simulink model "Flyback_with_comparator"  (R2016a)
settings: Solver=VariableStepAuto  StartTime=0.0  StopTime=0.5  RelTol=1e-3
libraries: powerlib x9, powerlib_meascontrol x1
settings Model: Creator=Mac  LastModifiedBy=Hp

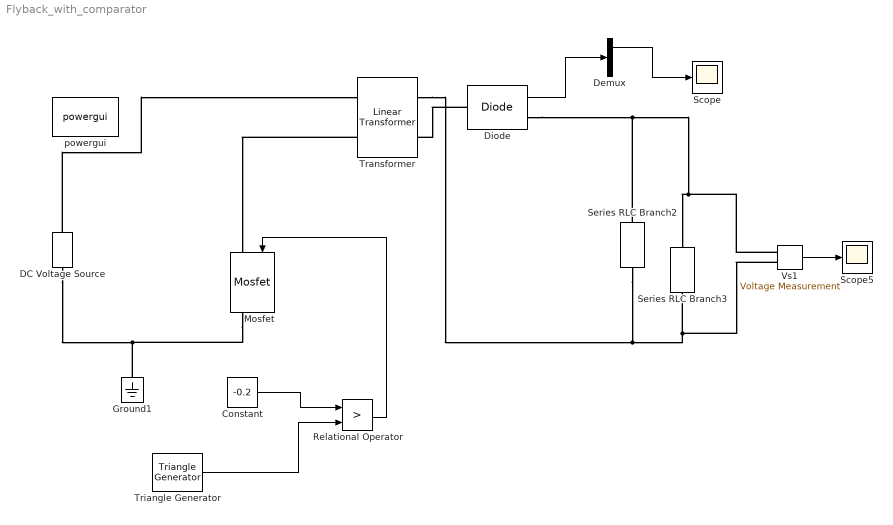
== system Flyback_with_comparator ==
  Constant : Constant  Value=-0.2
  DC Voltage Source : powerlib/Electrical Sources/DC Voltage Source  Amplitude=12  Measurements=None
  Demux : Demux  Outputs=2
  Diode : powerlib/Power Electronics/Diode  Ron=0.001  Lon=0  Vf=0.8  IC=0  UseSnubber=off  Rs=500  Cs=250e-9  Measurements=on
  Ground1 : powerlib/Elements/Ground  LConnTagsString=a
  Mosfet : powerlib/Power Electronics/Mosfet  Ron=0.00001  Lon=0  Rd=0.01  Vfd=0  IC=0  Rs=1e5  Cs=inf  Measurements=on
  Relational Operator : RelationalOperator  Operator=>  OutDataTypeStr=boolean
  Scope : Scope
  Scope5 : Scope
  Series RLC Branch2 : powerlib/Elements/Series RLC Branch  LConnTagsString=__new0  RConnTagsString=__new0  BranchType=C  Resistance=25.6  Inductance=200e-3  SetiL0=off  InitialCurrent=0  Capacitance=100e-6  Setx0=off  InitialVoltage=0  Measurements=Branch voltage
  Series RLC Branch3 : powerlib/Elements/Series RLC Branch  LConnTagsString=__new0  RConnTagsString=__new0  BranchType=R  Resistance=25.6  Inductance=200e-3  SetiL0=off  InitialCurrent=0  Capacitance=1e-6  Setx0=off  InitialVoltage=0  Measurements=Branch voltage
  Transformer : powerlib/Elements/Linear Transformer  UNITS=SI  NominalPower=[ 1000 100e3 ]  winding1=[500 0 0]  winding2=[3000 0 0]  ThreeWindings=off  winding3=[3.15e+05 315.06 8.8673e-08]  RmLm=[100000 14.4e-6]  Measurements=All voltages and currents  DataType=on
  Triangle Generator : powerlib_meascontrol/Pulse & Signal Generators/Triangle Generator  Freq=100e3  Phase=90  Ts=0
  Vs1 : powerlib/Measurements/Voltage Measurement  PhasorSimulation=off  OutputType=Complex  PSBequivalent=0
  "powergui " : powerlib/powergui  Priority=1  SimulationMode=Continuous  SolverType=Tustin/Backward Euler (TBE)  SampleTime=1e-7  frequency=60  SPID=on  DisableSnubberDevices=off  DisableRonSwitches=on  DisableVfSwitches=on  SwTol=0  DisplayEquations=off  Interpol=off  ExternalGateDelay=off  methode=off  Ts=10  FunctionMessages=off  echomessages=off  HookPort=off  EnableUseOfTLC=off  x0status=blocks  frequencyindice=0  Pbase=100e6  ErrMax=1e-4  Iterations=50  UnitsV=kV  UnitsW=MW  buscounter=0  RestoreLinks=warning  ResistiveCurrentMeasurement=off  Frange=[0:2:500]  Ylog=off  Xlog=on  ShowGrid=off  save=off  variable=ZData  structure=0  ZoomFFT=off  StartTime=0.0  cycles=1  DisplayStyle=1  fundamental=60  FreqAxis=off  MaxFrequency=1000  frequencyindicesteady=1  RmsSteady=1  display=off
  wires:
  Vs1/1 -> Scope5/1
  Constant/1 -> Relational Operator/1
  Triangle Generator/1 -> Relational Operator/2
  Relational Operator/1 -> Mosfet/1
  Diode/1 -> Demux/1
  Demux/1 -> Scope/1
  connections:
  Transformer/RConn1 -- Series RLC Branch2/RConn1 -- Vs1/LConn2 -- Series RLC Branch3/RConn1
  Vs1/LConn1 -- Series RLC Branch2/LConn1 -- Diode/RConn1 -- Series RLC Branch3/LConn1
  Transformer/LConn2 -- Mosfet/LConn1
  DC Voltage Source/RConn1 -- Transformer/LConn1
  Diode/LConn1 -- Transformer/RConn2
  DC Voltage Source/LConn1 -- Mosfet/RConn1 -- Ground1/LConn1
